simulink model "Tavola3_bis_FL"  (R2018b)
settings: Solver=VariableStepAuto  StartTime=0.0  StopTime=10.0  RelTol=1e-3
settings Model: Creator=Utente  LastModifiedBy=giga4

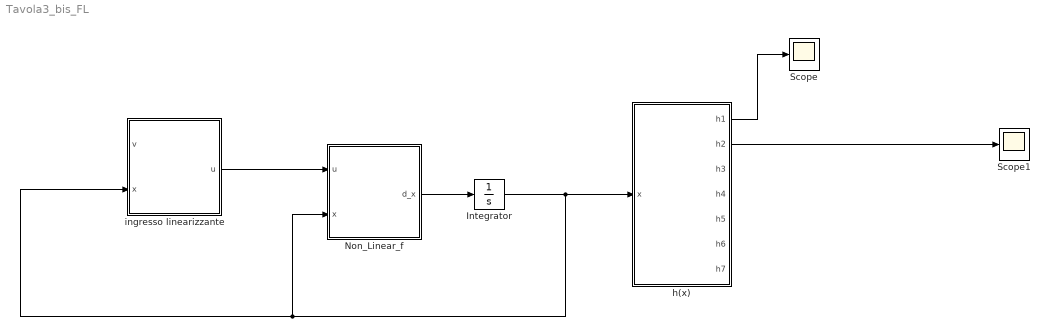
== system Tavola3_bis_FL ==
  Integrator : Integrator  InitialCondition=[0,0,0,pi/180,0,5,.5]
  "Non_Linear_f " : MATLAB Function  TreatAsAtomicUnit=on
  Scope : Scope
  Scope1 : Scope
  h(x) : MATLAB Function  TreatAsAtomicUnit=on
  ingresso linearizzante : MATLAB Function  TreatAsAtomicUnit=on
  wires:
  "Non_Linear_f "/1(d_x) -> Integrator/1
  Integrator/1 -> ingresso linearizzante/2(x), "Non_Linear_f "/2(x), h(x)/1(x)
  h(x)/1(h1) -> Scope/1
  h(x)/2(h2) -> Scope1/1
  ingresso linearizzante/1(u) -> "Non_Linear_f "/1(u)

== matlab function Tavola3_bis_FL/h(x) ==
  data: x input; h1 output; h2 output; h3 output; h4 output; h5 output; h6 output; h7 output
function [h1,h2,h3,h4,h5,h6,h7] = h(x)

x1 = x(1);
x2 = x(2);
x3 = x(3);
x4 = x(4);
x5 = x(5);
x6 = x(6);
x7 = x(7);


h1 = x1;
h2 = x2;
h3 = x3;
h4 = x4;
h5 = x5;
h6 = x6;
h7 = x7;

== matlab function Tavola3_bis_FL/Non_Linear_f  ==
  data: u input; d_x output; x input
function d_x = statespacef(u,x)

x1 = x(1);
x2 = x(2);
x3 = x(3);
x4 = x(4);
x5 = x(5);
x6 = x(6);
x7 = x(7);


f =                                                                                                                               [x6*cos(x3);
                                                                                                                                  x6*sin(x3);
                                                                                                                                          x7;
                                                                                                                                          x5;
 (2.39*sin(2.0*x4)*x5^2)/(4.79*cos(x4)^2 - 12.5) - (173.0*sin(x4))/(4.79*cos(x4)^2 - 12.5) - (3.28*x7^2*sin(2.0*x4))/(4.79*cos(x4)^2 - 12.5);
       (1.99*sin(3.0*x4) - 6.77*sin(x4))*x7^2 + (23.5*sin(2.0*x4))/(4.79*cos(x4)^2 - 12.5) - (2.19*x5^2*sin(2.0*x4))/(4.79*cos(x4)^2 - 12.5);
                                       (0.547*x6*x7*sin(x4))/(0.228*cos(x4)^2 - 0.315) + (0.228*x5*x7*sin(2.0*x4))/(0.228*cos(x4)^2 - 0.315)];
                                   
g1 =                        [0;
                             0;
                             0;
                             0;
      (35*cos(x3))/16 + 249/80;
 - (35*cos(x4))/64 - 1603/1600;
                             0];
g2 = [0;0;0;0;0;0;1];

d_x = f + [g1,g2]*u;

== matlab function Tavola3_bis_FL/ingresso linearizzante ==
  data: v input; u output; x input
function u = inputLinearizzante(v,x)

x1 = x(1);
x2 = x(2);
x3 = x(3);
x4 = x(4);
x5 = x(5);
x6 = x(6);
x7 = x(7);

inv_E = [ -(0.0967*(33.0*cos(x4)^2 - 86.0)*(500.0*x6*cos(x3) + 2000.0*x7*sin(3.0*x4)*sin(x3) - 6777.0*x7*sin(x3)*sin(x4)))/(1.66e4*x7^2*sin(3.0*x4)*cos(x3)^2 + 1.66e4*x7^2*sin(3.0*x4)*sin(x3)^2 - 5.64e4*x7^2*cos(x3)^2*sin(x4) - 5.64e4*x7^2*sin(x3)^2*sin(x4) + 9077.0*x7^2*sin(3.0*x4)*cos(x4)*sin(x3)^2 + 4555.0*x5*x6*sin(2.0*x4)*cos(x3)^2 + 3200.0*x5*x6*sin(2.0*x4)*cos(x3)^3 + 4555.0*x5*x6*sin(2.0*x4)*sin(x3)^2 - 3.08e4*x7^2*cos(x3)^2*cos(x4)*sin(x4) - 3.08e4*x7^2*cos(x4)*sin(x3)^2*sin(x4) - 6388.0*x7^2*sin(3.0*x4)*cos(x3)^2*cos(x4)^2 - 3488.0*x7^2*sin(3.0*x4)*cos(x3)^2*cos(x4)^3 - 6388.0*x7^2*sin(3.0*x4)*cos(x4)^2*sin(x3)^2 - 3488.0*x7^2*sin(3.0*x4)*cos(x4)^3*sin(x3)^2 + 2.16e4*x7^2*cos(x3)^2*cos(x4)^2*sin(x4) + 1.18e4*x7^2*cos(x3)^2*cos(x4)^3*sin(x4) + 2.16e4*x7^2*cos(x4)^2*sin(x3)^2*sin(x4) + 1.18e4*x7^2*cos(x4)^3*sin(x3)^2*sin(x4) + 9077.0*x7^2*sin(3.0*x4)*cos(x3)^2*cos(x4) + 3200.0*x5*x6*sin(2.0*x4)*cos(x3)*sin(x3)^2),                                                                      -(0.0967*(33.0*cos(x4)^2 - 86.0)*(500.0*x6*sin(x3) - 2000.0*x7*sin(3.0*x4)*cos(x3) + 6777.0*x7*cos(x3)*sin(x4)))/(1.66e4*x7^2*sin(3.0*x4)*cos(x3)^2 + 1.66e4*x7^2*sin(3.0*x4)*sin(x3)^2 - 5.64e4*x7^2*cos(x3)^2*sin(x4) - 5.64e4*x7^2*sin(x3)^2*sin(x4) + 9077.0*x7^2*sin(3.0*x4)*cos(x4)*sin(x3)^2 + 4555.0*x5*x6*sin(2.0*x4)*cos(x3)^2 + 3200.0*x5*x6*sin(2.0*x4)*cos(x3)^3 + 4555.0*x5*x6*sin(2.0*x4)*sin(x3)^2 - 3.08e4*x7^2*cos(x3)^2*cos(x4)*sin(x4) - 3.08e4*x7^2*cos(x4)*sin(x3)^2*sin(x4) - 6388.0*x7^2*sin(3.0*x4)*cos(x3)^2*cos(x4)^2 - 3488.0*x7^2*sin(3.0*x4)*cos(x3)^2*cos(x4)^3 - 6388.0*x7^2*sin(3.0*x4)*cos(x4)^2*sin(x3)^2 - 3488.0*x7^2*sin(3.0*x4)*cos(x4)^3*sin(x3)^2 + 2.16e4*x7^2*cos(x3)^2*cos(x4)^2*sin(x4) + 1.18e4*x7^2*cos(x3)^2*cos(x4)^3*sin(x4) + 2.16e4*x7^2*cos(x4)^2*sin(x3)^2*sin(x4) + 1.18e4*x7^2*cos(x4)^3*sin(x3)^2*sin(x4) + 9077.0*x7^2*sin(3.0*x4)*cos(x3)^2*cos(x4) + 3200.0*x5*x6*sin(2.0*x4)*cos(x3)*sin(x3)^2);
          -(5.0e-4*(9.09e6*x5*sin(2.0*x4)*sin(x3) - 8.33e6*x7*cos(x3) - 4.55e6*x7*cos(x3)*cos(x4) + 3.2e6*x7*cos(x3)*cos(x4)^2 + 1.74e6*x7*cos(x3)*cos(x4)^3 + 6.39e6*x5*sin(2.0*x4)*cos(x3)*sin(x3)))/(1.66e4*x7^2*sin(3.0*x4)*cos(x3)^2 + 1.66e4*x7^2*sin(3.0*x4)*sin(x3)^2 - 5.64e4*x7^2*cos(x3)^2*sin(x4) - 5.64e4*x7^2*sin(x3)^2*sin(x4) + 9077.0*x7^2*sin(3.0*x4)*cos(x4)*sin(x3)^2 + 4555.0*x5*x6*sin(2.0*x4)*cos(x3)^2 + 3200.0*x5*x6*sin(2.0*x4)*cos(x3)^3 + 4555.0*x5*x6*sin(2.0*x4)*sin(x3)^2 - 3.08e4*x7^2*cos(x3)^2*cos(x4)*sin(x4) - 3.08e4*x7^2*cos(x4)*sin(x3)^2*sin(x4) - 6388.0*x7^2*sin(3.0*x4)*cos(x3)^2*cos(x4)^2 - 3488.0*x7^2*sin(3.0*x4)*cos(x3)^2*cos(x4)^3 - 6388.0*x7^2*sin(3.0*x4)*cos(x4)^2*sin(x3)^2 - 3488.0*x7^2*sin(3.0*x4)*cos(x4)^3*sin(x3)^2 + 2.16e4*x7^2*cos(x3)^2*cos(x4)^2*sin(x4) + 1.18e4*x7^2*cos(x3)^2*cos(x4)^3*sin(x4) + 2.16e4*x7^2*cos(x4)^2*sin(x3)^2*sin(x4) + 1.18e4*x7^2*cos(x4)^3*sin(x3)^2*sin(x4) + 9077.0*x7^2*sin(3.0*x4)*cos(x3)^2*cos(x4) + 3200.0*x5*x6*sin(2.0*x4)*cos(x3)*sin(x3)^2), (5.0e-4*(8.33e6*x7*sin(x3) + 9.09e6*x5*sin(2.0*x4)*cos(x3) + 6.39e6*x5*sin(2.0*x4)*cos(x3)^2 + 4.55e6*x7*cos(x4)*sin(x3) - 3.2e6*x7*cos(x4)^2*sin(x3) - 1.74e6*x7*cos(x4)^3*sin(x3)))/(1.66e4*x7^2*sin(3.0*x4)*cos(x3)^2 + 1.66e4*x7^2*sin(3.0*x4)*sin(x3)^2 - 5.64e4*x7^2*cos(x3)^2*sin(x4) - 5.64e4*x7^2*sin(x3)^2*sin(x4) + 9077.0*x7^2*sin(3.0*x4)*cos(x4)*sin(x3)^2 + 4555.0*x5*x6*sin(2.0*x4)*cos(x3)^2 + 3200.0*x5*x6*sin(2.0*x4)*cos(x3)^3 + 4555.0*x5*x6*sin(2.0*x4)*sin(x3)^2 - 3.08e4*x7^2*cos(x3)^2*cos(x4)*sin(x4) - 3.08e4*x7^2*cos(x4)*sin(x3)^2*sin(x4) - 6388.0*x7^2*sin(3.0*x4)*cos(x3)^2*cos(x4)^2 - 3488.0*x7^2*sin(3.0*x4)*cos(x3)^2*cos(x4)^3 - 6388.0*x7^2*sin(3.0*x4)*cos(x4)^2*sin(x3)^2 - 3488.0*x7^2*sin(3.0*x4)*cos(x4)^3*sin(x3)^2 + 2.16e4*x7^2*cos(x3)^2*cos(x4)^2*sin(x4) + 1.18e4*x7^2*cos(x3)^2*cos(x4)^3*sin(x4) + 2.16e4*x7^2*cos(x4)^2*sin(x3)^2*sin(x4) + 1.18e4*x7^2*cos(x4)^3*sin(x3)^2*sin(x4) + 9077.0*x7^2*sin(3.0*x4)*cos(x3)^2*cos(x4) + 3200.0*x5*x6*sin(2.0*x4)*cos(x3)*sin(x3)^2)];
 
Gamma =   [x5*cos(x3)*(x7^2*(5.98*cos(3.0*x4) - 6.77*cos(x4)) + (46.9*cos(2.0*x4))/(4.79*cos(x4)^2 - 12.5) - (4.38*x5^2*cos(2.0*x4))/(4.79*cos(x4)^2 - 12.5) + (225.0*sin(2.0*x4)*cos(x4)*sin(x4))/(4.79*cos(x4)^2 - 12.5)^2 - (21.0*x5^2*sin(2.0*x4)*cos(x4)*sin(x4))/(4.79*cos(x4)^2 - 12.5)^2) - 1.0*((0.547*x6*x7*sin(x4))/(0.228*cos(x4)^2 - 0.315) + (0.228*x5*x7*sin(2.0*x4))/(0.228*cos(x4)^2 - 0.315))*(x6*sin(x3) - 2.0*x7*cos(x3)*(1.99*sin(3.0*x4) - 6.77*sin(x4))) - 1.0*x7*sin(x3)*((1.99*sin(3.0*x4) - 6.77*sin(x4))*x7^2 + (23.5*sin(2.0*x4))/(4.79*cos(x4)^2 - 12.5) - (2.19*x5^2*sin(2.0*x4))/(4.79*cos(x4)^2 - 12.5)) - 1.0*x7*(sin(x3)*((1.99*sin(3.0*x4) - 6.77*sin(x4))*x7^2 + (23.5*sin(2.0*x4))/(4.79*cos(x4)^2 - 12.5) - (2.19*x5^2*sin(2.0*x4))/(4.79*cos(x4)^2 - 12.5)) + x6*x7*cos(x3)) + (4.38*x5*sin(2.0*x4)*cos(x3)*((3.28*sin(2.0*x4)*x7^2)/(4.79*cos(x4)^2 - 12.5) + (173.0*sin(x4))/(4.79*cos(x4)^2 - 12.5) - (2.39*x5^2*sin(2.0*x4))/(4.79*cos(x4)^2 - 12.5)))/(4.79*cos(x4)^2 - 12.5);
         ((0.547*x6*x7*sin(x4))/(0.228*cos(x4)^2 - 0.315) + (0.228*x5*x7*sin(2.0*x4))/(0.228*cos(x4)^2 - 0.315))*(x6*cos(x3) + 2.0*x7*sin(x3)*(1.99*sin(3.0*x4) - 6.77*sin(x4))) + x7*(cos(x3)*((1.99*sin(3.0*x4) - 6.77*sin(x4))*x7^2 + (23.5*sin(2.0*x4))/(4.79*cos(x4)^2 - 12.5) - (2.19*x5^2*sin(2.0*x4))/(4.79*cos(x4)^2 - 12.5)) - 1.0*x6*x7*sin(x3)) + x5*sin(x3)*(x7^2*(5.98*cos(3.0*x4) - 6.77*cos(x4)) + (46.9*cos(2.0*x4))/(4.79*cos(x4)^2 - 12.5) - (4.38*x5^2*cos(2.0*x4))/(4.79*cos(x4)^2 - 12.5) + (225.0*sin(2.0*x4)*cos(x4)*sin(x4))/(4.79*cos(x4)^2 - 12.5)^2 - (21.0*x5^2*sin(2.0*x4)*cos(x4)*sin(x4))/(4.79*cos(x4)^2 - 12.5)^2) + x7*cos(x3)*((1.99*sin(3.0*x4) - 6.77*sin(x4))*x7^2 + (23.5*sin(2.0*x4))/(4.79*cos(x4)^2 - 12.5) - (2.19*x5^2*sin(2.0*x4))/(4.79*cos(x4)^2 - 12.5)) + (4.38*x5*sin(2.0*x4)*sin(x3)*((3.28*sin(2.0*x4)*x7^2)/(4.79*cos(x4)^2 - 12.5) + (173.0*sin(x4))/(4.79*cos(x4)^2 - 12.5) - (2.39*x5^2*sin(2.0*x4))/(4.79*cos(x4)^2 - 12.5)))/(4.79*cos(x4)^2 - 12.5)];
  
u = -inv_E*Gamma+inv_E*v;
